simulink model "DataPath"  (R2025a)
settings: Solver=FixedStepAuto  StartTime=0  StopTime=0.02  FixedStep=1e-7  RelTol=1e-3
undefined symbols (not defined in the file): Bit_1, Bit_2, Bit_3, Bit_4, Bit_5, Bit_6, Bit_7, Bit_8
libraries: simulink_extras x126, fl_lib x34, nesl_utility x18, simulink x2
(part 4 of 7)

== system DataPath/Subsystem/ALU_REG/Subsystem1 ==
  Data : Inport
  Store : Inport  Port=2
  Clock : Inport  Port=3
  Clear : Inport  Port=4
  AND : Logic  IconShape=distinctive  AllPortsSameDT=off  OutDataTypeStr=boolean
  AND1 : Logic  IconShape=distinctive  AllPortsSameDT=off  OutDataTypeStr=boolean
  D Flip-Flop : simulink_extras/Flip Flops/D Flip-Flop
  NOT : Logic  Operator=NOT  IconShape=distinctive  AllPortsSameDT=off  OutDataTypeStr=boolean
  NOT1 : Logic  Operator=NOT  IconShape=distinctive  AllPortsSameDT=off  OutDataTypeStr=boolean
  OR : Logic  Operator=OR  IconShape=distinctive  AllPortsSameDT=off  OutDataTypeStr=boolean
  Q : Outport
  !Q : Outport  Port=2
  wires:
  AND1/1 -> OR/2
  AND/1 -> OR/1
  D Flip-Flop/1 -> Q/1, AND1/2
  NOT/1 -> AND1/1
  Store/1 -> AND/2, NOT/1
  Clock/1 -> D Flip-Flop/2
  Data/1 -> AND/1
  OR/1 -> D Flip-Flop/1
  D Flip-Flop/2 -> !Q/1
  Clear/1 -> NOT1/1
  NOT1/1 -> D Flip-Flop/3

== system DataPath/Subsystem/ALU_REG/Subsystem3 ==
  Data : Inport
  Store : Inport  Port=2
  Clock : Inport  Port=3
  Clear : Inport  Port=4
  AND : Logic  IconShape=distinctive  AllPortsSameDT=off  OutDataTypeStr=boolean
  AND1 : Logic  IconShape=distinctive  AllPortsSameDT=off  OutDataTypeStr=boolean
  D Flip-Flop : simulink_extras/Flip Flops/D Flip-Flop
  NOT : Logic  Operator=NOT  IconShape=distinctive  AllPortsSameDT=off  OutDataTypeStr=boolean
  NOT1 : Logic  Operator=NOT  IconShape=distinctive  AllPortsSameDT=off  OutDataTypeStr=boolean
  OR : Logic  Operator=OR  IconShape=distinctive  AllPortsSameDT=off  OutDataTypeStr=boolean
  Q : Outport
  !Q : Outport  Port=2
  wires:
  AND1/1 -> OR/2
  AND/1 -> OR/1
  D Flip-Flop/1 -> Q/1, AND1/2
  NOT/1 -> AND1/1
  Store/1 -> AND/2, NOT/1
  Clock/1 -> D Flip-Flop/2
  Data/1 -> AND/1
  OR/1 -> D Flip-Flop/1
  D Flip-Flop/2 -> !Q/1
  Clear/1 -> NOT1/1
  NOT1/1 -> D Flip-Flop/3

== system DataPath/Subsystem/Add Subtract Logic/Subsystem1 ==
  AND : Inport
  OR : Inport  Port=2
  XOR : Inport  Port=3
  !A : Inport  Port=4
  "!B " : Inport  Port=5
  SR : Inport  Port=6
  SL : Inport  Port=7
  OR1 : Logic  Operator=OR  Inputs=4  IconShape=distinctive  AllPortsSameDT=off  OutDataTypeStr=boolean
  OR2 : Logic  Operator=OR  Inputs=4  IconShape=distinctive  AllPortsSameDT=off  OutDataTypeStr=boolean
  OR3 : Logic  Operator=OR  Inputs=4  IconShape=distinctive  AllPortsSameDT=off  OutDataTypeStr=boolean
  C : Outport
  B : Outport  Port=2
  "A " : Outport  Port=3
  wires:
  OR2/1 -> C/1
  OR1/1 -> B/1
  OR3/1 -> "A "/1
  OR/1 -> OR3/1
  XOR/1 -> OR3/2, OR2/3
  !A/1 -> OR3/3, OR1/3
  "!B "/1 -> OR3/4, OR1/4, OR2/4
  SR/1 -> OR2/1
  SL/1 -> OR1/1
  AND/1 -> OR1/2, OR2/2

== system DataPath/Subsystem/Add Subtract Logic/Subsystem2 ==
  LO : Inport
  Enable : Inport  Port=2
  C : Inport  Port=3
  B : Inport  Port=4
  A : Inport  Port=5
  AND{6..17} (12 alike) : Logic  IconShape=distinctive  AllPortsSameDT=off  OutDataTypeStr=boolean
  NOT1 : Logic  Operator=NOT  IconShape=distinctive  AllPortsSameDT=off  OutDataTypeStr=boolean
  NOT2 : Logic  Operator=NOT  IconShape=distinctive  AllPortsSameDT=off  OutDataTypeStr=boolean
  NOT3 : Logic  Operator=NOT  IconShape=distinctive  AllPortsSameDT=off  OutDataTypeStr=boolean
  S-R Flip-Flop : simulink_extras/Flip Flops/S-R Flip-Flop  initial_condition=0
  S-R Flip-Flop1 : simulink_extras/Flip Flops/S-R Flip-Flop  initial_condition=0
  S-R Flip-Flop2 : simulink_extras/Flip Flops/S-R Flip-Flop  initial_condition=0
  A Stored : Outport
  B Stored : Outport  Port=2
  C Stored : Outport  Port=3
  wires:
  AND6/1 -> NOT3/1, AND14/2
  AND8/1 -> AND10/2, NOT1/1
  AND12/1 -> S-R Flip-Flop1/2
  NOT3/1 -> AND11/2
  Enable/1 -> AND8/1, AND7/1, AND6/1, AND13/1, AND12/1, AND11/1, AND10/1, AND9/1, AND14/1
  AND14/1 -> S-R Flip-Flop/1
  AND10/1 -> S-R Flip-Flop2/1
  S-R Flip-Flop1/1 -> AND16/1  "Data"
  AND7/1 -> AND9/2, NOT2/1
  AND11/1 -> S-R Flip-Flop/2
  B/1 -> AND7/2
  LO/1 -> AND17/2, AND16/2, AND15/2
  AND13/1 -> S-R Flip-Flop2/2
  AND17/1 -> C Stored/1
  A/1 -> AND6/2
  NOT2/1 -> AND12/2
  AND16/1 -> B Stored/1
  NOT1/1 -> AND13/2
  AND15/1 -> A Stored/1
  S-R Flip-Flop2/1 -> AND17/1  "Data"
  AND9/1 -> S-R Flip-Flop1/1
  S-R Flip-Flop/1 -> AND15/1  "Data"
  C/1 -> AND8/2

== system DataPath/Subsystem/Normalize Div/Subsystem1 ==
  Data : Inport
  CLK : Inport  Port=2
  NOT9 : Logic  Operator=NOT  IconShape=distinctive  AllPortsSameDT=off  OutDataTypeStr=boolean
  Subsystem6 : Subsystem
  Subsystem7 : Subsystem
  !Q : Outport
  Q : Outport  Port=2
  wires:
  Subsystem7/1(Q) -> Subsystem6/1(Data)
  Subsystem6/1(Q) -> Q/1
  CLK/1 -> Subsystem6/2(CLK), NOT9/1
  NOT9/1 -> Subsystem7/2(CLK)
  Data/1 -> Subsystem7/1(Data)
  Subsystem6/2(!Q) -> !Q/1

== system DataPath/Subsystem/Normalize Div/Subsystem8 ==
  Data : Inport
  CLK : Inport  Port=2
  NOT9 : Logic  Operator=NOT  IconShape=distinctive  AllPortsSameDT=off  OutDataTypeStr=boolean
  Subsystem6 : Subsystem
  Subsystem7 : Subsystem
  !Q : Outport
  Q : Outport  Port=2
  wires:
  Subsystem7/1(Q) -> Subsystem6/1(Data)
  Subsystem6/1(Q) -> Q/1
  NOT9/1 -> Subsystem7/2(CLK)
  Data/1 -> Subsystem7/1(Data)
  Subsystem6/2(!Q) -> !Q/1
  CLK/1 -> Subsystem6/2(CLK), NOT9/1

== system DataPath/Subsystem/Stepper/Subsystem1 ==
  "Step_{n-1}" : Inport
  CLK : Inport  Port=2
  "OR_{n+1}" : Inport  Port=3
  AND1 : Logic  IconShape=distinctive  AllPortsSameDT=off  OutDataTypeStr=boolean
  DFF : Subsystem
  Delay : Delay  DelayLength=1  InputProcessing=Columns as channels (frame based)  SampleTime=1e-6
  NOT1 : Logic  Operator=NOT  IconShape=distinctive  AllPortsSameDT=off  OutDataTypeStr=boolean
  OR1 : Logic  Operator=OR  IconShape=distinctive  AllPortsSameDT=off  OutDataTypeStr=boolean
  "Step_{n}" : Outport
  "!Step_{n}" : Outport  Port=2
  "OR_{n}" : Outport  Port=3
  wires:
  NOT1/1 -> "!Step_{n}"/1, AND1/2
  CLK/1 -> DFF/2(CLK)
  AND1/1 -> DFF/1(Data)
  "OR_{n+1}"/1 -> OR1/2
  "Step_{n-1}"/1 -> AND1/1
  DFF/1(Q) -> "Step_{n}"/1, OR1/1
  OR1/1 -> Delay/1
  Delay/1 -> "OR_{n}"/1, NOT1/1

== system DataPath/Subsystem/Stepper/Subsystem2 ==
  "Step_{n-1}" : Inport
  CLK : Inport  Port=2
  "OR_{n+1}" : Inport  Port=3
  AND1 : Logic  IconShape=distinctive  AllPortsSameDT=off  OutDataTypeStr=boolean
  DFF : Subsystem
  Delay : Delay  DelayLength=1  InputProcessing=Columns as channels (frame based)  SampleTime=1e-6
  Delay One Step : Delay  DelayLength=1
  Delay One Step1 : Delay  DelayLength=1
  NOT1 : Logic  Operator=NOT  IconShape=distinctive  AllPortsSameDT=off  OutDataTypeStr=boolean
  OR1 : Logic  Operator=OR  IconShape=distinctive  AllPortsSameDT=off  OutDataTypeStr=boolean
  "Step_{n}" : Outport
  "!Step_{n}" : Outport  Port=2
  "OR_{n}" : Outport  Port=3
  wires:
  Delay One Step1/1 -> "!Step_{n}"/1, AND1/2
  CLK/1 -> DFF/2(CLK)
  AND1/1 -> DFF/1(Data)
  "OR_{n+1}"/1 -> OR1/2
  "Step_{n-1}"/1 -> AND1/1
  DFF/1(Q) -> "Step_{n}"/1, OR1/1
  OR1/1 -> Delay/1
  Delay/1 -> Delay One Step/1, NOT1/1
  Delay One Step/1 -> "OR_{n}"/1
  NOT1/1 -> Delay One Step1/1

== system DataPath/Subsystem/Stepper/Subsystem3 ==
  "Step_{n-1}" : Inport
  CLK : Inport  Port=2
  "OR_{n+1}" : Inport  Port=3
  AND1 : Logic  IconShape=distinctive  AllPortsSameDT=off  OutDataTypeStr=boolean
  DFF : Subsystem
  Delay : Delay  DelayLength=1  InputProcessing=Columns as channels (frame based)  SampleTime=1e-6
  NOT1 : Logic  Operator=NOT  IconShape=distinctive  AllPortsSameDT=off  OutDataTypeStr=boolean
  OR1 : Logic  Operator=OR  IconShape=distinctive  AllPortsSameDT=off  OutDataTypeStr=boolean
  "Step_{n}" : Outport
  "!Step_{n}" : Outport  Port=2
  "OR_{n}" : Outport  Port=3
  wires:
  NOT1/1 -> "!Step_{n}"/1, AND1/2
  CLK/1 -> DFF/2(CLK)
  AND1/1 -> DFF/1(Data)
  "OR_{n+1}"/1 -> OR1/2
  "Step_{n-1}"/1 -> AND1/1
  DFF/1(Q) -> "Step_{n}"/1, OR1/1
  OR1/1 -> Delay/1
  Delay/1 -> "OR_{n}"/1, NOT1/1

== system DataPath/Subsystem/Stepper/Subsystem4 ==
  "Step_{n-1}" : Inport
  CLK : Inport  Port=2
  "OR_{n+1}" : Inport  Port=3
  AND1 : Logic  IconShape=distinctive  AllPortsSameDT=off  OutDataTypeStr=boolean
  DFF : Subsystem
  Delay : Delay  DelayLength=1  InputProcessing=Columns as channels (frame based)  SampleTime=1e-6
  NOT1 : Logic  Operator=NOT  IconShape=distinctive  AllPortsSameDT=off  OutDataTypeStr=boolean
  OR1 : Logic  Operator=OR  IconShape=distinctive  AllPortsSameDT=off  OutDataTypeStr=boolean
  "Step_{n}" : Outport
  "!Step_{n}" : Outport  Port=2
  "OR_{n}" : Outport  Port=3
  wires:
  NOT1/1 -> "!Step_{n}"/1, AND1/2
  CLK/1 -> DFF/2(CLK)
  AND1/1 -> DFF/1(Data)
  "OR_{n+1}"/1 -> OR1/2
  "Step_{n-1}"/1 -> AND1/1
  DFF/1(Q) -> "Step_{n}"/1, OR1/1
  OR1/1 -> Delay/1
  Delay/1 -> "OR_{n}"/1, NOT1/1

== system DataPath/Subsystem/Subsystem1/Subsystem ==
  Out A1-LO : Inport
  Out A1-Mult : Inport  Port=2
  Out A1-CD : Inport  Port=3
  Out A1-ND : Inport  Port=4
  Out A1-SDR : Inport  Port=5
  OR : Logic  Operator=OR  Inputs=5  IconShape=distinctive  AllPortsSameDT=off  OutDataTypeStr=boolean
  Out A1 : Outport
  wires:
  Out A1-LO/1 -> OR/5
  Out A1-Mult/1 -> OR/1
  OR/1 -> Out A1/1  "Out A1"
  Out A1-CD/1 -> OR/2
  Out A1-ND/1 -> OR/3
  Out A1-SDR/1 -> OR/4

== system DataPath/Subsystem/Subsystem1/Subsystem10 ==
  LSB-Mult : Inport
  LSB-CD : Inport  Port=2
  OR2 : Logic  Operator=OR  IconShape=distinctive  AllPortsSameDT=off  OutDataTypeStr=boolean
  LSB : Outport
  wires:
  LSB-CD/1 -> OR2/1
  LSB-Mult/1 -> OR2/2
  OR2/1 -> LSB/1  "LSB"

== system DataPath/Subsystem/Subsystem1/Subsystem11 ==
  NegA-ND : Inport
  NegA-SDR : Inport  Port=2
  OR1 : Logic  Operator=OR  IconShape=distinctive  AllPortsSameDT=off  OutDataTypeStr=boolean
  NegA : Outport
  wires:
  NegA-ND/1 -> OR1/1
  NegA-SDR/1 -> OR1/2
  OR1/1 -> NegA/1  "Bus Switch"

== system DataPath/Subsystem/Subsystem1/Subsystem13 ==
  Store B2-Mult : Inport
  Store B2-CD : Inport  Port=2
  Store B2-SDR : Inport  Port=3
  CLR : Inport  Port=4
  OR2 : Logic  Operator=OR  Inputs=4  IconShape=distinctive  AllPortsSameDT=off  OutDataTypeStr=boolean
  Store B2 : Outport
  wires:
  Store B2-CD/1 -> OR2/2
  OR2/1 -> Store B2/1  "Store B2"
  Store B2-SDR/1 -> OR2/3
  Store B2-Mult/1 -> OR2/1
  CLR/1 -> OR2/4

== system DataPath/Subsystem/Subsystem1/Subsystem14 ==
  Store B1-ICS : Inport
  Store B1-Mult : Inport  Port=2
  Store B1-ND : Inport  Port=3
  In4 : Inport  Port=4
  OR1 : Logic  Operator=OR  Inputs=4  IconShape=distinctive  AllPortsSameDT=off  OutDataTypeStr=boolean
  Store B1 : Outport
  wires:
  Store B1-ND/1 -> OR1/2
  Store B1-ICS/1 -> OR1/1
  OR1/1 -> Store B1/1  "Store B1"
  Store B1-Mult/1 -> OR1/3
  In4/1 -> OR1/4

== system DataPath/Subsystem/Subsystem1/Subsystem2 ==
  Out B2-Mult : Inport
  Out B2-CD : Inport  Port=2
  Out B2-SDR : Inport  Port=3
  OR2 : Logic  Operator=OR  Inputs=3  IconShape=distinctive  AllPortsSameDT=off  OutDataTypeStr=boolean
  Out B2 : Outport
  wires:
  Out B2-Mult/1 -> OR2/1
  Out B2-CD/1 -> OR2/2
  Out B2-SDR/1 -> OR2/3
  OR2/1 -> Out B2/1  "Out B2"

== system DataPath/Subsystem/Subsystem1/Subsystem3 ==
  Out ALU-LO : Inport
  Out ALU-Mult : Inport  Port=2
  Out ALU-ND : Inport  Port=3
  Out ALU-CD : Inport  Port=4
  Out ALU-SDR : Inport  Port=5
  OR3 : Logic  Operator=OR  Inputs=5  IconShape=distinctive  AllPortsSameDT=off  OutDataTypeStr=boolean
  Out ALU : Outport
  wires:
  Out ALU-SDR/1 -> OR3/4
  Out ALU-Mult/1 -> OR3/1
  OR3/1 -> Out ALU/1  "Out A1"
  Out ALU-LO/1 -> OR3/5
  Out ALU-ND/1 -> OR3/3
  Out ALU-CD/1 -> OR3/2

== system DataPath/Subsystem/Subsystem1/Subsystem5 ==
  Out B1-LO : Inport
  Out B1-mult : Inport  Port=2
  Out B1-CD : Inport  Port=3
  Out B1-ND : Inport  Port=4
  OR1 : Logic  Operator=OR  Inputs=4  IconShape=distinctive  AllPortsSameDT=off  OutDataTypeStr=boolean
  Out B1 : Outport
  wires:
  Out B1-CD/1 -> OR1/2
  Out B1-mult/1 -> OR1/1
  Out B1-LO/1 -> OR1/4
  OR1/1 -> Out B1/1  "Out B1"
  Out B1-ND/1 -> OR1/3

== system DataPath/Subsystem/Subsystem1/Subsystem6 ==
  Store A1-ICS : Inport
  Store A1-ND : Inport  Port=2
  Store A1-CD : Inport  Port=3
  Store A1-SDR : Inport  Port=4
  CLR : Inport  Port=5
  OR : Logic  Operator=OR  Inputs=5  IconShape=distinctive  AllPortsSameDT=off  OutDataTypeStr=boolean
  Store A1 : Outport
  wires:
  Store A1-CD/1 -> OR/2
  OR/1 -> Store A1/1  "Store A1"
  Store A1-ICS/1 -> OR/1
  Store A1-ND/1 -> OR/3
  Store A1-SDR/1 -> OR/4
  CLR/1 -> OR/5

== system DataPath/Subsystem/Subsystem1/Subsystem7 ==
  ADD ND : Inport
  ADD CD : Inport  Port=2
  ADD-SDR : Inport  Port=3
  OR1 : Logic  Operator=OR  Inputs=3  IconShape=distinctive  AllPortsSameDT=off  OutDataTypeStr=boolean
  "ADD " : Outport
  wires:
  ADD ND/1 -> OR1/2
  ADD CD/1 -> OR1/1
  OR1/1 -> "ADD "/1
  ADD-SDR/1 -> OR1/3

== system DataPath/Subsystem/Subsystem1/Subsystem9 ==
  Out DP-LO : Inport
  Out DP-Mult : Inport  Port=2
  Out DP-Div : Inport  Port=3
  OR3 : Logic  Operator=OR  Inputs=3  IconShape=distinctive  AllPortsSameDT=off  OutDataTypeStr=boolean
  Out DP : Outport
  wires:
  OR3/1 -> Out DP/1
  Out DP-Mult/1 -> OR3/2
  Out DP-Div/1 -> OR3/3
  Out DP-LO/1 -> OR3/1

== system DataPath/Subsystem1/ALU/ALU MUX ==
  note: Each Enabler is a set of 8 tri-state buffers
  0/0/0 : Inport
  0/0/1 : Inport  Port=2
  0/1/0 : Inport  Port=3
  0/1/1 : Inport  Port=4
  1/0/0 : Inport  Port=5
  1/0/1 : Inport  Port=6
  1/1/0 : Inport  Port=7
  1/1/1 : Inport  Port=8
  Bus1 : Inport  Port=9
  Bus2 : Inport  Port=10
  Bus3 : Inport  Port=11
  Bus4 : Inport  Port=12
  Bus5 : Inport  Port=13
  Bus6 : Inport  Port=14
  Bus7 : Inport  Port=15
  Bus8 : Inport  Port=16
  Delay One Step1 : Delay  DelayLength=1
  Delay One Step3 : Delay  DelayLength=1
  MATLAB Function1 : MATLAB Function  TreatAsAtomicUnit=on
  MATLAB Function2 : MATLAB Function  TreatAsAtomicUnit=on
  MATLAB Function3 : MATLAB Function  TreatAsAtomicUnit=on
  MATLAB Function4 : MATLAB Function  TreatAsAtomicUnit=on
  MATLAB Function5 : MATLAB Function  TreatAsAtomicUnit=on
  MATLAB Function6 : MATLAB Function  TreatAsAtomicUnit=on
  MATLAB Function7 : MATLAB Function  TreatAsAtomicUnit=on
  MATLAB Function8 : MATLAB Function  TreatAsAtomicUnit=on
  Mux : Mux  Inputs=8
  Mux1 : Mux  Inputs=8
  ALU Output : Outport
  wires:
  1/1/1/1 -> Mux/8
  1/1/0/1 -> Mux/7
  1/0/1/1 -> Mux/6
  1/0/0/1 -> Mux/5
  0/1/1/1 -> Mux/4
  0/1/0/1 -> Mux/3
  0/0/1/1 -> Mux/2
  0/0/0/1 -> Mux/1
  Bus3/1 -> MATLAB Function2/1(InputBus)
  Bus5/1 -> MATLAB Function4/1(InputBus)
  Bus8/1 -> MATLAB Function8/1(InputBus)
  Bus2/1 -> MATLAB Function6/1(InputBus)
  Bus4/1 -> MATLAB Function3/1(InputBus)
  Bus1/1 -> MATLAB Function1/1(InputBus)
  Bus6/1 -> MATLAB Function5/1(InputBus)
  Bus7/1 -> MATLAB Function7/1(InputBus)
  Mux/1 -> MATLAB Function8/2(Selection), MATLAB Function7/2(Selection), MATLAB Function5/2(Selection), MATLAB Function4/2(Selection), MATLAB Function3/2(Selection), MATLAB Function2/2(Selection), MATLAB Function1/2(Selection), MATLAB Function6/2(Selection)
  MATLAB Function6/1(output) -> Mux1/2
  MATLAB Function2/1(output) -> Mux1/3
  MATLAB Function3/1(output) -> Mux1/4
  MATLAB Function4/1(output) -> Mux1/5
  MATLAB Function5/1(output) -> Mux1/6
  MATLAB Function7/1(output) -> Mux1/7
  MATLAB Function8/1(output) -> Mux1/8
  MATLAB Function1/1(output) -> Mux1/1
  Mux1/1 -> Delay One Step1/1
  Delay One Step1/1 -> ALU Output/1

== system DataPath/Subsystem1/ALU/Adder & Logic Module ==
  Subtract mode : Inport
  Neg_A : Inport  Port=2
  Bus_A : Inport  Port=3
  Bus_B : Inport  Port=4
  Constant : Constant
  Constant1 : Constant  Value=0
  Delay One Step1 : Delay  DelayLength=1
  Delay One Step3 : Delay  DelayLength=1
  Demux1 : Demux  Outputs=8
  Demux2 : Demux  Outputs=8
  Display1 : Display
  Display3 : Display
  MATLAB Function1 : MATLAB Function  TreatAsAtomicUnit=on
  MATLAB Function3 : MATLAB Function  TreatAsAtomicUnit=on
  Subsystem1 : Subsystem
      settings: PortSchema="{\"entries\":[{\"content\":{\"sides\":[{\"content\":{\"connectorIds\":[\"In1\",\"In2\",\"Out3\",\"Out4\"]},\"type\":\"ConnectorPlacement.EquallySpacedRectSide\",\"uuid\":\"d566efe6-1fc5-4e96-a6c3-64a47f89d9c9\"},{\"content\":{\"connectorIds\":[\"Out1\",\"In6\",\"In7\"],\"side\":\"RIGHT\"},\"type\":\"ConnectorPlacement.EquallySpacedRectSide\",\"uuid\":\"006cd780-973d-4bae-abc8-89f745b28566\"},{\"content\":{\"connectorIds\":[\"In3\",\"In4\"],\"side\":\"TOP\"},\"type\":\"ConnectorPlacement.EquallySpacedRectSide\",\"uuid\":\"c760ecb1-3a5c-4ba0-9224-1c9b5ce710fd\"},{\"content\":{\"connectorIds\":[\"In5\",\"Out2\"],\"side\":\"BOTTOM\"},\"type\":\"ConnectorPlacement.EquallySpacedRectSide\",\"uuid\":\"178f6c5d-529f-4f0d-80ca-fb6729cf398e\"}]},\"type\":\"ConnectorPlacement.EquallySpacedConnector\",\"uuid\":\"d5293939-72db-46a2-88f3-163e4f70d202\"}],\"packageUris\":[\"http://schema.mathworks.com/mf0/Connector/R2020b\"],\"version\":\"1.0\"}"
  Subsystem2 : Subsystem
      settings: PortSchema="{\"entries\":[{\"content\":{\"sides\":[{\"content\":{\"connectorIds\":[\"In1\",\"In2\",\"Out3\",\"Out4\"]},\"type\":\"ConnectorPlacement.EquallySpacedRectSide\",\"uuid\":\"d566efe6-1fc5-4e96-a6c3-64a47f89d9c9\"},{\"content\":{\"connectorIds\":[\"Out1\",\"In6\",\"In7\"],\"side\":\"RIGHT\"},\"type\":\"ConnectorPlacement.EquallySpacedRectSide\",\"uuid\":\"006cd780-973d-4bae-abc8-89f745b28566\"},{\"content\":{\"connectorIds\":[\"In3\",\"In4\"],\"side\":\"TOP\"},\"type\":\"ConnectorPlacement.EquallySpacedRectSide\",\"uuid\":\"c760ecb1-3a5c-4ba0-9224-1c9b5ce710fd\"},{\"content\":{\"connectorIds\":[\"In5\",\"Out2\"],\"side\":\"BOTTOM\"},\"type\":\"ConnectorPlacement.EquallySpacedRectSide\",\"uuid\":\"178f6c5d-529f-4f0d-80ca-fb6729cf398e\"}]},\"type\":\"ConnectorPlacement.EquallySpacedConnector\",\"uuid\":\"d5293939-72db-46a2-88f3-163e4f70d202\"}],\"packageUris\":[\"http://schema.mathworks.com/mf0/Connector/R2020b\"],\"version\":\"1.0\"}"
  Subsystem3 : Subsystem
      settings: PortSchema="{\"entries\":[{\"content\":{\"sides\":[{\"content\":{\"connectorIds\":[\"In1\",\"In2\",\"Out3\",\"Out4\"]},\"type\":\"ConnectorPlacement.EquallySpacedRectSide\",\"uuid\":\"d566efe6-1fc5-4e96-a6c3-64a47f89d9c9\"},{\"content\":{\"connectorIds\":[\"Out1\",\"In6\",\"In7\"],\"side\":\"RIGHT\"},\"type\":\"ConnectorPlacement.EquallySpacedRectSide\",\"uuid\":\"006cd780-973d-4bae-abc8-89f745b28566\"},{\"content\":{\"connectorIds\":[\"In3\",\"In4\"],\"side\":\"TOP\"},\"type\":\"ConnectorPlacement.EquallySpacedRectSide\",\"uuid\":\"c760ecb1-3a5c-4ba0-9224-1c9b5ce710fd\"},{\"content\":{\"connectorIds\":[\"In5\",\"Out2\"],\"side\":\"BOTTOM\"},\"type\":\"ConnectorPlacement.EquallySpacedRectSide\",\"uuid\":\"178f6c5d-529f-4f0d-80ca-fb6729cf398e\"}]},\"type\":\"ConnectorPlacement.EquallySpacedConnector\",\"uuid\":\"d5293939-72db-46a2-88f3-163e4f70d202\"}],\"packageUris\":[\"http://schema.mathworks.com/mf0/Connector/R2020b\"],\"version\":\"1.0\"}"
  Subsystem4 : Subsystem
      settings: PortSchema="{\"entries\":[{\"content\":{\"sides\":[{\"content\":{\"connectorIds\":[\"In1\",\"In2\",\"Out3\",\"Out4\"]},\"type\":\"ConnectorPlacement.EquallySpacedRectSide\",\"uuid\":\"d566efe6-1fc5-4e96-a6c3-64a47f89d9c9\"},{\"content\":{\"connectorIds\":[\"Out1\",\"In6\",\"In7\"],\"side\":\"RIGHT\"},\"type\":\"ConnectorPlacement.EquallySpacedRectSide\",\"uuid\":\"006cd780-973d-4bae-abc8-89f745b28566\"},{\"content\":{\"connectorIds\":[\"In3\",\"In4\"],\"side\":\"TOP\"},\"type\":\"ConnectorPlacement.EquallySpacedRectSide\",\"uuid\":\"c760ecb1-3a5c-4ba0-9224-1c9b5ce710fd\"},{\"content\":{\"connectorIds\":[\"In5\",\"Out2\"],\"side\":\"BOTTOM\"},\"type\":\"ConnectorPlacement.EquallySpacedRectSide\",\"uuid\":\"178f6c5d-529f-4f0d-80ca-fb6729cf398e\"}]},\"type\":\"ConnectorPlacement.EquallySpacedConnector\",\"uuid\":\"d5293939-72db-46a2-88f3-163e4f70d202\"}],\"packageUris\":[\"http://schema.mathworks.com/mf0/Connector/R2020b\"],\"version\":\"1.0\"}"
  Subsystem5 : Subsystem
      settings: PortSchema="{\"entries\":[{\"content\":{\"sides\":[{\"content\":{\"connectorIds\":[\"In1\",\"In2\",\"Out3\",\"Out4\"]},\"type\":\"ConnectorPlacement.EquallySpacedRectSide\",\"uuid\":\"d566efe6-1fc5-4e96-a6c3-64a47f89d9c9\"},{\"content\":{\"connectorIds\":[\"Out1\",\"In6\",\"In7\"],\"side\":\"RIGHT\"},\"type\":\"ConnectorPlacement.EquallySpacedRectSide\",\"uuid\":\"006cd780-973d-4bae-abc8-89f745b28566\"},{\"content\":{\"connectorIds\":[\"In3\",\"In4\"],\"side\":\"TOP\"},\"type\":\"ConnectorPlacement.EquallySpacedRectSide\",\"uuid\":\"c760ecb1-3a5c-4ba0-9224-1c9b5ce710fd\"},{\"content\":{\"connectorIds\":[\"In5\",\"Out2\"],\"side\":\"BOTTOM\"},\"type\":\"ConnectorPlacement.EquallySpacedRectSide\",\"uuid\":\"178f6c5d-529f-4f0d-80ca-fb6729cf398e\"}]},\"type\":\"ConnectorPlacement.EquallySpacedConnector\",\"uuid\":\"d5293939-72db-46a2-88f3-163e4f70d202\"}],\"packageUris\":[\"http://schema.mathworks.com/mf0/Connector/R2020b\"],\"version\":\"1.0\"}"
  Subsystem6 : Subsystem
      settings: PortSchema="{\"entries\":[{\"content\":{\"sides\":[{\"content\":{\"connectorIds\":[\"In1\",\"In2\",\"Out3\",\"Out4\"]},\"type\":\"ConnectorPlacement.EquallySpacedRectSide\",\"uuid\":\"d566efe6-1fc5-4e96-a6c3-64a47f89d9c9\"},{\"content\":{\"connectorIds\":[\"Out1\",\"In6\",\"In7\"],\"side\":\"RIGHT\"},\"type\":\"ConnectorPlacement.EquallySpacedRectSide\",\"uuid\":\"006cd780-973d-4bae-abc8-89f745b28566\"},{\"content\":{\"connectorIds\":[\"In3\",\"In4\"],\"side\":\"TOP\"},\"type\":\"ConnectorPlacement.EquallySpacedRectSide\",\"uuid\":\"c760ecb1-3a5c-4ba0-9224-1c9b5ce710fd\"},{\"content\":{\"connectorIds\":[\"In5\",\"Out2\"],\"side\":\"BOTTOM\"},\"type\":\"ConnectorPlacement.EquallySpacedRectSide\",\"uuid\":\"178f6c5d-529f-4f0d-80ca-fb6729cf398e\"}]},\"type\":\"ConnectorPlacement.EquallySpacedConnector\",\"uuid\":\"d5293939-72db-46a2-88f3-163e4f70d202\"}],\"packageUris\":[\"http://schema.mathworks.com/mf0/Connector/R2020b\"],\"version\":\"1.0\"}"
  Subsystem7 : Subsystem
      settings: PortSchema="{\"entries\":[{\"content\":{\"sides\":[{\"content\":{\"connectorIds\":[\"In1\",\"In2\",\"Out3\",\"Out4\"]},\"type\":\"ConnectorPlacement.EquallySpacedRectSide\",\"uuid\":\"d566efe6-1fc5-4e96-a6c3-64a47f89d9c9\"},{\"content\":{\"connectorIds\":[\"Out1\",\"In6\",\"In7\"],\"side\":\"RIGHT\"},\"type\":\"ConnectorPlacement.EquallySpacedRectSide\",\"uuid\":\"006cd780-973d-4bae-abc8-89f745b28566\"},{\"content\":{\"connectorIds\":[\"In3\",\"In4\"],\"side\":\"TOP\"},\"type\":\"ConnectorPlacement.EquallySpacedRectSide\",\"uuid\":\"c760ecb1-3a5c-4ba0-9224-1c9b5ce710fd\"},{\"content\":{\"connectorIds\":[\"In5\",\"Out2\"],\"side\":\"BOTTOM\"},\"type\":\"ConnectorPlacement.EquallySpacedRectSide\",\"uuid\":\"178f6c5d-529f-4f0d-80ca-fb6729cf398e\"}]},\"type\":\"ConnectorPlacement.EquallySpacedConnector\",\"uuid\":\"d5293939-72db-46a2-88f3-163e4f70d202\"}],\"packageUris\":[\"http://schema.mathworks.com/mf0/Connector/R2020b\"],\"version\":\"1.0\"}"
  Subsystem8 : Subsystem
      settings: PortSchema="{\"entries\":[{\"content\":{\"sides\":[{\"content\":{\"connectorIds\":[\"In1\",\"In2\",\"Out3\",\"Out4\"]},\"type\":\"ConnectorPlacement.EquallySpacedRectSide\",\"uuid\":\"d566efe6-1fc5-4e96-a6c3-64a47f89d9c9\"},{\"content\":{\"connectorIds\":[\"Out1\",\"In6\",\"In7\"],\"side\":\"RIGHT\"},\"type\":\"ConnectorPlacement.EquallySpacedRectSide\",\"uuid\":\"006cd780-973d-4bae-abc8-89f745b28566\"},{\"content\":{\"connectorIds\":[\"In3\",\"In4\"],\"side\":\"TOP\"},\"type\":\"ConnectorPlacement.EquallySpacedRectSide\",\"uuid\":\"c760ecb1-3a5c-4ba0-9224-1c9b5ce710fd\"},{\"content\":{\"connectorIds\":[\"In5\",\"Out2\"],\"side\":\"BOTTOM\"},\"type\":\"ConnectorPlacement.EquallySpacedRectSide\",\"uuid\":\"178f6c5d-529f-4f0d-80ca-fb6729cf398e\"}]},\"type\":\"ConnectorPlacement.EquallySpacedConnector\",\"uuid\":\"d5293939-72db-46a2-88f3-163e4f70d202\"}],\"packageUris\":[\"http://schema.mathworks.com/mf0/Connector/R2020b\"],\"version\":\"1.0\"}"
  Bus1 : Outport
  Bus2 : Outport  Port=2
  Bus3 : Outport  Port=3
  Bus4 : Outport  Port=4
  Bus5 : Outport  Port=5
  Bus6 : Outport  Port=6
  Bus7 : Outport  Port=7
  Bus8 : Outport  Port=8
  A=B : Outport  Port=9
  A>B : Outport  Port=10
  Overflow : Outport  Port=11
  wires:
  Subsystem8/1(Carry Out) -> Subsystem2/2(Carry In)
  Subsystem6/1(Carry Out) -> Subsystem5/2(Carry In)
  Subsystem3/1(Carry Out) -> Subsystem6/2(Carry In)
  Subsystem8/2(Bus) -> Bus8/1
  Subsystem7/2(Bus) -> Bus1/1
  Subsystem4/2(Bus) -> Bus2/1
  Subsystem5/2(Bus) -> Bus3/1
  Subsystem6/2(Bus) -> Bus4/1
  Subsystem3/2(Bus) -> Bus5/1
  Subsystem1/2(Bus) -> Bus6/1
  Subsystem2/2(Bus) -> Bus7/1
  Subtract mode/1 -> Subsystem8/2(Carry In), Subsystem8/5(Subtract), Subsystem7/5(Subtract), Subsystem2/5(Subtract), Subsystem4/5(Subtract), Subsystem1/5(Subtract), Subsystem5/5(Subtract), Subsystem6/5(Subtract), Subsystem3/5(Subtract)
  Subsystem7/1(Carry Out) -> Overflow/1
  Bus_A/1 -> Delay One Step3/1  "Bus A"
  MATLAB Function1/1(Decimal) -> Display1/1
  Bus_B/1 -> Delay One Step1/1  "Bus B"
  MATLAB Function3/1(Decimal) -> Display3/1
  Subsystem2/1(Carry Out) -> Subsystem1/2(Carry In)
  Subsystem1/1(Carry Out) -> Subsystem3/2(Carry In)
  Subsystem5/1(Carry Out) -> Subsystem4/2(Carry In)
  Subsystem4/1(Carry Out) -> Subsystem7/2(Carry In)
  Neg_A/1 -> Subsystem8/1(Neg_A), Subsystem2/1(Neg_A), Subsystem1/1(Neg_A), Subsystem6/1(Neg_A), Subsystem5/1(Neg_A), Subsystem4/1(Neg_A), Subsystem7/1(Neg_A), Subsystem3/1(Neg_A)
  Delay One Step3/1 -> MATLAB Function1/1(Binary), Demux2/1
  Delay One Step1/1 -> MATLAB Function3/1(Binary), Demux1/1
  Demux1/1 -> Subsystem7/3(B)
  Demux1/2 -> Subsystem4/3(B)
  Demux1/3 -> Subsystem5/3(B)
  Demux1/4 -> Subsystem6/3(B)
  Demux1/5 -> Subsystem3/3(B)
  Demux1/6 -> Subsystem1/3(B)
  Demux1/7 -> Subsystem2/3(B)
  Demux1/8 -> Subsystem8/3(B)
  Demux2/8 -> Subsystem8/4(A)
  Demux2/7 -> Subsystem2/4(A)
  Demux2/6 -> Subsystem1/4(A)
  Demux2/5 -> Subsystem3/4(A)
  Demux2/4 -> Subsystem6/4(A)
  Demux2/3 -> Subsystem5/4(A)
  Demux2/2 -> Subsystem4/4(A)
  Demux2/1 -> Subsystem7/4(A)
  Subsystem7/3(A >B Next) -> Subsystem4/6(A>B Prev)
  Subsystem7/4(= Currently) -> Subsystem4/7(= So far)
  Subsystem4/4(= Currently) -> Subsystem5/7(= So far)
  Subsystem4/3(A >B Next) -> Subsystem5/6(A>B Prev)
  Subsystem5/4(= Currently) -> Subsystem6/7(= So far)
  Subsystem5/3(A >B Next) -> Subsystem6/6(A>B Prev)
  Constant/1 -> Subsystem7/7(= So far)
  Subsystem1/3(= Currently) -> Subsystem2/6(= So far)
  Subsystem1/4(A >B Next) -> Subsystem2/7(A>B Prev)
  Subsystem3/4(A >B Next) -> Subsystem1/7(A>B Prev)
  Subsystem3/3(= Currently) -> Subsystem1/6(= So far)
  Subsystem2/4(A >B Next) -> Subsystem8/7(A>B Prev)
  Subsystem2/3(= Currently) -> Subsystem8/6(= So far)
  Subsystem8/4(A >B Next) -> A>B/1
  Subsystem8/3(= Currently) -> A=B/1
  Subsystem6/4(= Currently) -> Subsystem3/6(= So far)
  Subsystem6/3(A >B Next) -> Subsystem3/7(A>B Prev)
  Constant1/1 -> Subsystem7/6(A>B Prev)

== system DataPath/Subsystem1/ALU/FlagAndDecode ==
  note: A/B/C
  SM : Inport
  Sel_A : Inport  Port=2
  Sel_B : Inport  Port=3
  Sel_C : Inport  Port=4
  ALU Bus : Inport  Port=5
  Overflow : Inport  Port=6
  AND1 : Logic  IconShape=distinctive  AllPortsSameDT=off  OutDataTypeStr=boolean
  AND{3..10} (8 alike) : Logic  Inputs=3  IconShape=distinctive  AllPortsSameDT=off  OutDataTypeStr=boolean
  AND2 : Logic  IconShape=distinctive  AllPortsSameDT=off  OutDataTypeStr=boolean
  Demux1 : Demux  Outputs=8
  NAND : Logic  Operator=NAND  IconShape=distinctive  AllPortsSameDT=off  OutDataTypeStr=boolean
  NOR1 : Logic  Operator=NOR  Inputs=8  IconShape=distinctive  AllPortsSameDT=off  OutDataTypeStr=boolean
  NOT{,1..3} (4 alike) : Logic  Operator=NOT  IconShape=distinctive  AllPortsSameDT=off  OutDataTypeStr=boolean
  0/0/0 : Outport
  0/0/1 : Outport  Port=2
  0/1/0 : Outport  Port=3
  0/1/1 : Outport  Port=4
  1/0/0 : Outport  Port=5
  1/0/1 : Outport  Port=6
  1/1/0 : Outport  Port=7
  1/1/1 : Outport  Port=8
  Zero : Outport  Port=9
  Negative : Outport  Port=10
  wires:
  SM/1 -> AND2/1, NOT/1
  Demux1/1 -> NOR1/1, AND2/2
  NOT/1 -> NAND/2
  Demux1/4 -> NOR1/4
  NOR1/1 -> AND1/2  "Byte_zero"
  Overflow/1 -> NAND/1
  Demux1/5 -> NOR1/5
  NAND/1 -> AND1/1  "No_Overflow"
  Demux1/8 -> NOR1/8
  Demux1/6 -> NOR1/6
  ALU Bus/1 -> Demux1/1
  Demux1/7 -> NOR1/7
  Demux1/3 -> NOR1/3
  AND1/1 -> Zero/1  "Zero"
  AND2/1 -> Negative/1
  Demux1/2 -> NOR1/2
  AND3/1 -> 0/0/0/1
  NOT1/1 -> AND6/1, AND5/1, AND4/1, AND3/1
  AND9/1 -> 1/1/0/1
  Sel_C/1 -> AND10/3, AND8/3, AND6/3, AND4/3, NOT3/1
  AND7/1 -> 1/0/0/1
  AND6/1 -> 0/1/1/1
  NOT2/1 -> AND4/2, AND7/2, AND8/2, AND3/2
  Sel_B/1 -> AND10/2, AND9/2, AND6/2, AND5/2, NOT2/1
  AND4/1 -> 0/0/1/1
  NOT3/1 -> AND9/3, AND7/3, AND5/3, AND3/3
  Sel_A/1 -> AND10/1, AND9/1, AND8/1, AND7/1, NOT1/1
  AND5/1 -> 0/1/0/1
  AND8/1 -> 1/0/1/1
  AND10/1 -> 1/1/1/1

== system DataPath/Subsystem1/ALU Regs/A1 ==
  Data bus : Inport
  Store : Inport  Port=2
  CLK : Inport  Port=3
  Demux : Demux  Outputs=8
  Mux : Mux  Inputs=8
  Subsystem1 : Subsystem
  Subsystem2 : Subsystem
  Subsystem3 : Subsystem
  Subsystem4 : Subsystem
  Subsystem5 : Subsystem
  Subsystem6 : Subsystem
  Subsystem7 : Subsystem
  Subsystem8 : Subsystem
  "Q Bus " : Outport
  wires:
  Demux/4 -> Subsystem2/1(Data)
  Mux/1 -> "Q Bus "/1
  Demux/2 -> Subsystem1/1(Data)
  Data bus/1 -> Demux/1
  Subsystem6/1(Q) -> Mux/8
  Store/1 -> Subsystem1/2(Store), Subsystem4/2(Store), Subsystem2/2(Store), Subsystem7/2(Store), Subsystem5/2(Store), Subsystem6/2(Store), Subsystem8/2(Store), Subsystem3/2(Store)
  Demux/5 -> Subsystem7/1(Data)
  Demux/7 -> Subsystem8/1(Data)
  Demux/3 -> Subsystem4/1(Data)
  Subsystem7/1(Q) -> Mux/5
  Demux/6 -> Subsystem5/1(Data)
  Subsystem1/1(Q) -> Mux/2
  Demux/1 -> Subsystem3/1(Data)
  Subsystem3/1(Q) -> Mux/1
  Demux/8 -> Subsystem6/1(Data)
  Subsystem8/1(Q) -> Mux/7
  Subsystem2/1(Q) -> Mux/4
  Subsystem4/1(Q) -> Mux/3
  Subsystem5/1(Q) -> Mux/6
  CLK/1 -> Subsystem1/3(Clock), Subsystem4/3(Clock), Subsystem2/3(Clock), Subsystem7/3(Clock), Subsystem5/3(Clock), Subsystem6/3(Clock), Subsystem8/3(Clock), Subsystem3/3(Clock)

== system DataPath/Subsystem1/ALU Regs/A2 ==
  Data bus : Inport
  Store : Inport  Port=2
  CLK : Inport  Port=3
  Demux : Demux  Outputs=8
  Mux : Mux  Inputs=8
  Subsystem1 : Subsystem
  Subsystem2 : Subsystem
  Subsystem3 : Subsystem
  Subsystem4 : Subsystem
  Subsystem5 : Subsystem
  Subsystem6 : Subsystem
  Subsystem7 : Subsystem
  Subsystem8 : Subsystem
  "Q Bus " : Outport
  wires:
  Demux/4 -> Subsystem2/1(Data)
  Mux/1 -> "Q Bus "/1
  Demux/2 -> Subsystem1/1(Data)
  Data bus/1 -> Demux/1
  Subsystem6/1(Q) -> Mux/8
  Store/1 -> Subsystem1/2(Store), Subsystem4/2(Store), Subsystem2/2(Store), Subsystem7/2(Store), Subsystem5/2(Store), Subsystem6/2(Store), Subsystem8/2(Store), Subsystem3/2(Store)
  Demux/5 -> Subsystem7/1(Data)
  Demux/7 -> Subsystem8/1(Data)
  Demux/3 -> Subsystem4/1(Data)
  Subsystem7/1(Q) -> Mux/5
  Demux/6 -> Subsystem5/1(Data)
  Subsystem1/1(Q) -> Mux/2
  Demux/1 -> Subsystem3/1(Data)
  Subsystem3/1(Q) -> Mux/1
  Demux/8 -> Subsystem6/1(Data)
  Subsystem8/1(Q) -> Mux/7
  Subsystem2/1(Q) -> Mux/4
  Subsystem4/1(Q) -> Mux/3
  Subsystem5/1(Q) -> Mux/6
  CLK/1 -> Subsystem1/3(Clock), Subsystem4/3(Clock), Subsystem2/3(Clock), Subsystem7/3(Clock), Subsystem5/3(Clock), Subsystem6/3(Clock), Subsystem8/3(Clock), Subsystem3/3(Clock)

== system DataPath/Subsystem1/ALU Regs/B1 ==
  Data bus : Inport
  Store : Inport  Port=2
  CLK : Inport  Port=3
  Demux : Demux  Outputs=8
  Mux : Mux  Inputs=8
  Subsystem1 : Subsystem
  Subsystem2 : Subsystem
  Subsystem3 : Subsystem
  Subsystem4 : Subsystem
  Subsystem5 : Subsystem
  Subsystem6 : Subsystem
  Subsystem7 : Subsystem
  Subsystem8 : Subsystem
  "Q Bus " : Outport
  wires:
  Demux/4 -> Subsystem2/1(Data)
  Mux/1 -> "Q Bus "/1
  Demux/2 -> Subsystem1/1(Data)
  Data bus/1 -> Demux/1
  Subsystem6/1(Q) -> Mux/8
  Store/1 -> Subsystem1/2(Store), Subsystem4/2(Store), Subsystem2/2(Store), Subsystem7/2(Store), Subsystem5/2(Store), Subsystem6/2(Store), Subsystem8/2(Store), Subsystem3/2(Store)
  Demux/5 -> Subsystem7/1(Data)
  Demux/7 -> Subsystem8/1(Data)
  Demux/3 -> Subsystem4/1(Data)
  Subsystem7/1(Q) -> Mux/5
  Demux/6 -> Subsystem5/1(Data)
  Subsystem1/1(Q) -> Mux/2
  Demux/1 -> Subsystem3/1(Data)
  Subsystem3/1(Q) -> Mux/1
  Demux/8 -> Subsystem6/1(Data)
  Subsystem8/1(Q) -> Mux/7
  Subsystem2/1(Q) -> Mux/4
  Subsystem4/1(Q) -> Mux/3
  Subsystem5/1(Q) -> Mux/6
  CLK/1 -> Subsystem1/3(Clock), Subsystem4/3(Clock), Subsystem2/3(Clock), Subsystem7/3(Clock), Subsystem5/3(Clock), Subsystem6/3(Clock), Subsystem8/3(Clock), Subsystem3/3(Clock)

== system DataPath/Subsystem1/ALU Regs/B2 ==
  Data bus : Inport
  Store : Inport  Port=2
  CLK : Inport  Port=3
  Demux : Demux  Outputs=8
  Mux : Mux  Inputs=8
  Subsystem1 : Subsystem
  Subsystem2 : Subsystem
  Subsystem3 : Subsystem
  Subsystem4 : Subsystem
  Subsystem5 : Subsystem
  Subsystem6 : Subsystem
  Subsystem7 : Subsystem
  Subsystem8 : Subsystem
  "Q Bus " : Outport
  wires:
  Demux/4 -> Subsystem2/1(Data)
  Mux/1 -> "Q Bus "/1
  Demux/2 -> Subsystem1/1(Data)
  Data bus/1 -> Demux/1
  Subsystem6/1(Q) -> Mux/8
  Store/1 -> Subsystem1/2(Store), Subsystem4/2(Store), Subsystem2/2(Store), Subsystem7/2(Store), Subsystem5/2(Store), Subsystem6/2(Store), Subsystem8/2(Store), Subsystem3/2(Store)
  Demux/5 -> Subsystem7/1(Data)
  Demux/7 -> Subsystem8/1(Data)
  Demux/3 -> Subsystem4/1(Data)
  Subsystem7/1(Q) -> Mux/5
  Demux/6 -> Subsystem5/1(Data)
  Subsystem1/1(Q) -> Mux/2
  Demux/1 -> Subsystem3/1(Data)
  Subsystem3/1(Q) -> Mux/1
  Demux/8 -> Subsystem6/1(Data)
  Subsystem8/1(Q) -> Mux/7
  Subsystem2/1(Q) -> Mux/4
  Subsystem4/1(Q) -> Mux/3
  Subsystem5/1(Q) -> Mux/6
  CLK/1 -> Subsystem1/3(Clock), Subsystem4/3(Clock), Subsystem2/3(Clock), Subsystem7/3(Clock), Subsystem5/3(Clock), Subsystem6/3(Clock), Subsystem8/3(Clock), Subsystem3/3(Clock)

== system DataPath/Subsystem1/ALU Regs/Subsystem2 ==
  Bus B1 : Inport
  B1 : Inport  Port=2
  B2 : Inport  Port=3
  Bus B 2 : Inport  Port=4
  Demux : Demux  Outputs=8
  Demux1 : Demux  Outputs=8
  MATLAB Function : MATLAB Function  TreatAsAtomicUnit=on
  Multiport Switch{,1..7} (8 alike) : MultiPortSwitch  DataPortOrder=Specify indices  Inputs=2  DataPortIndices={0,1,-1}  SaturateOnIntegerOverflow=off  InputSameDT=off
  Mux : Mux  Inputs=8
  Zero{,1..7} (8 alike) : Constant  Value=0  OutDataTypeStr=Inherit: Inherit via back propagation
  But Out : Outport
  wires:
  Demux1/7 -> Multiport Switch6/3
  Multiport Switch2/1 -> Mux/3
  Demux/4 -> Multiport Switch3/2
  Bus B 2/1 -> Demux1/1
  Multiport Switch6/1 -> Mux/7
  Demux1/1 -> Multiport Switch/3
  Multiport Switch3/1 -> Mux/4
  Zero/1 -> Multiport Switch/4
  MATLAB Function/1(Select) -> Multiport Switch7/1, Multiport Switch6/1, Multiport Switch5/1, Multiport Switch4/1, Multiport Switch3/1, Multiport Switch2/1, Multiport Switch1/1, Multiport Switch/1
  Demux/2 -> Multiport Switch1/2
  Demux/6 -> Multiport Switch5/2
  Demux/8 -> Multiport Switch7/2
  Multiport Switch/1 -> Mux/1
  Demux1/3 -> Multiport Switch2/3
  Zero6/1 -> Multiport Switch6/4
  Bus B1/1 -> Demux/1
  B2/1 -> MATLAB Function/2(A2)
  Zero5/1 -> Multiport Switch5/4
  Zero4/1 -> Multiport Switch4/4
  Demux/5 -> Multiport Switch4/2
  Zero2/1 -> Multiport Switch2/4
  Zero7/1 -> Multiport Switch7/4
  Demux1/4 -> Multiport Switch3/3
  Demux1/5 -> Multiport Switch4/3
  Multiport Switch5/1 -> Mux/6
  Multiport Switch1/1 -> Mux/2
  Demux1/2 -> Multiport Switch1/3
  Mux/1 -> But Out/1
  Zero3/1 -> Multiport Switch3/4
  Zero1/1 -> Multiport Switch1/4
  Demux/7 -> Multiport Switch6/2
  Demux1/8 -> Multiport Switch7/3
  Multiport Switch7/1 -> Mux/8
  Demux1/6 -> Multiport Switch5/3
  Demux/3 -> Multiport Switch2/2
  Multiport Switch4/1 -> Mux/5
  Demux/1 -> Multiport Switch/2
  B1/1 -> MATLAB Function/1(A1)

== system DataPath/Subsystem1/ALU Regs/Subsystem4 ==
  Bus A1 : Inport
  A1 : Inport  Port=2
  A2 : Inport  Port=3
  Bus A2 : Inport  Port=4
  Demux : Demux  Outputs=8
  Demux1 : Demux  Outputs=8
  MATLAB Function : MATLAB Function  TreatAsAtomicUnit=on
  Multiport Switch{,1..7} (8 alike) : MultiPortSwitch  DataPortOrder=Specify indices  Inputs=2  DataPortIndices={0,1,-1}  SaturateOnIntegerOverflow=off  InputSameDT=off
  Mux : Mux  Inputs=8
  Zero{,1..7} (8 alike) : Constant  Value=0  OutDataTypeStr=Inherit: Inherit via back propagation
  But Out : Outport
  wires:
  Demux1/7 -> Multiport Switch6/3
  Multiport Switch2/1 -> Mux/3
  Demux/4 -> Multiport Switch3/2
  Bus A2/1 -> Demux1/1
  Multiport Switch6/1 -> Mux/7
  Demux1/1 -> Multiport Switch/3
  Multiport Switch3/1 -> Mux/4
  Zero/1 -> Multiport Switch/4
  MATLAB Function/1(Select) -> Multiport Switch1/1, Multiport Switch7/1, Multiport Switch6/1, Multiport Switch5/1, Multiport Switch4/1, Multiport Switch3/1, Multiport Switch2/1, Multiport Switch/1
  Demux/2 -> Multiport Switch1/2
  Demux/6 -> Multiport Switch5/2
  Demux/8 -> Multiport Switch7/2
  Multiport Switch/1 -> Mux/1
  Demux1/3 -> Multiport Switch2/3
  Zero6/1 -> Multiport Switch6/4
  Bus A1/1 -> Demux/1
  A2/1 -> MATLAB Function/2(A2)
  Zero5/1 -> Multiport Switch5/4
  Zero4/1 -> Multiport Switch4/4
  Demux/5 -> Multiport Switch4/2
  Zero2/1 -> Multiport Switch2/4
  Zero7/1 -> Multiport Switch7/4
  Demux1/4 -> Multiport Switch3/3
  Demux1/5 -> Multiport Switch4/3
  Multiport Switch5/1 -> Mux/6
  Multiport Switch1/1 -> Mux/2
  Demux1/2 -> Multiport Switch1/3
  Mux/1 -> But Out/1
  Zero3/1 -> Multiport Switch3/4
  Zero1/1 -> Multiport Switch1/4
  Demux/7 -> Multiport Switch6/2
  Demux1/8 -> Multiport Switch7/3
  Multiport Switch7/1 -> Mux/8
  Demux1/6 -> Multiport Switch5/3
  Demux/3 -> Multiport Switch2/2
  Multiport Switch4/1 -> Mux/5
  Demux/1 -> Multiport Switch/2
  A1/1 -> MATLAB Function/1(A1)

== system DataPath/Subsystem1/ALU_REG/Subsystem1 ==
  Data : Inport
  Store : Inport  Port=2
  Clock : Inport  Port=3
  Clear : Inport  Port=4
  AND : Logic  IconShape=distinctive  AllPortsSameDT=off  OutDataTypeStr=boolean
  AND1 : Logic  IconShape=distinctive  AllPortsSameDT=off  OutDataTypeStr=boolean
  D Flip-Flop : simulink_extras/Flip Flops/D Flip-Flop
  NOT : Logic  Operator=NOT  IconShape=distinctive  AllPortsSameDT=off  OutDataTypeStr=boolean
  NOT1 : Logic  Operator=NOT  IconShape=distinctive  AllPortsSameDT=off  OutDataTypeStr=boolean
  OR : Logic  Operator=OR  IconShape=distinctive  AllPortsSameDT=off  OutDataTypeStr=boolean
  Q : Outport
  !Q : Outport  Port=2
  wires:
  AND1/1 -> OR/2
  AND/1 -> OR/1
  D Flip-Flop/1 -> Q/1, AND1/2
  NOT/1 -> AND1/1
  Store/1 -> AND/2, NOT/1
  Clock/1 -> D Flip-Flop/2
  Data/1 -> AND/1
  OR/1 -> D Flip-Flop/1
  D Flip-Flop/2 -> !Q/1
  Clear/1 -> NOT1/1
  NOT1/1 -> D Flip-Flop/3

== system DataPath/Subsystem1/ALU_REG/Subsystem3 ==
  Data : Inport
  Store : Inport  Port=2
  Clock : Inport  Port=3
  Clear : Inport  Port=4
  AND : Logic  IconShape=distinctive  AllPortsSameDT=off  OutDataTypeStr=boolean
  AND1 : Logic  IconShape=distinctive  AllPortsSameDT=off  OutDataTypeStr=boolean
  D Flip-Flop : simulink_extras/Flip Flops/D Flip-Flop
  NOT : Logic  Operator=NOT  IconShape=distinctive  AllPortsSameDT=off  OutDataTypeStr=boolean
  NOT1 : Logic  Operator=NOT  IconShape=distinctive  AllPortsSameDT=off  OutDataTypeStr=boolean
  OR : Logic  Operator=OR  IconShape=distinctive  AllPortsSameDT=off  OutDataTypeStr=boolean
  Q : Outport
  !Q : Outport  Port=2
  wires:
  AND1/1 -> OR/2
  AND/1 -> OR/1
  D Flip-Flop/1 -> Q/1, AND1/2
  NOT/1 -> AND1/1
  Store/1 -> AND/2, NOT/1
  Clock/1 -> D Flip-Flop/2
  Data/1 -> AND/1
  OR/1 -> D Flip-Flop/1
  D Flip-Flop/2 -> !Q/1
  Clear/1 -> NOT1/1
  NOT1/1 -> D Flip-Flop/3

== system DataPath/Subsystem1/Add Subtract Logic/Subsystem1 ==
  AND : Inport
  OR : Inport  Port=2
  XOR : Inport  Port=3
  !A : Inport  Port=4
  "!B " : Inport  Port=5
  SR : Inport  Port=6
  SL : Inport  Port=7
  OR1 : Logic  Operator=OR  Inputs=4  IconShape=distinctive  AllPortsSameDT=off  OutDataTypeStr=boolean
  OR2 : Logic  Operator=OR  Inputs=4  IconShape=distinctive  AllPortsSameDT=off  OutDataTypeStr=boolean
  OR3 : Logic  Operator=OR  Inputs=4  IconShape=distinctive  AllPortsSameDT=off  OutDataTypeStr=boolean
  C : Outport
  B : Outport  Port=2
  "A " : Outport  Port=3
  wires:
  OR2/1 -> C/1
  OR1/1 -> B/1
  OR3/1 -> "A "/1
  OR/1 -> OR3/1
  XOR/1 -> OR3/2, OR2/3
  !A/1 -> OR3/3, OR1/3
  "!B "/1 -> OR3/4, OR1/4, OR2/4
  SR/1 -> OR2/1
  SL/1 -> OR1/1
  AND/1 -> OR1/2, OR2/2

== system DataPath/Subsystem1/Add Subtract Logic/Subsystem2 ==
  LO : Inport
  Enable : Inport  Port=2
  C : Inport  Port=3
  B : Inport  Port=4
  A : Inport  Port=5
  AND{6..17} (12 alike) : Logic  IconShape=distinctive  AllPortsSameDT=off  OutDataTypeStr=boolean
  NOT1 : Logic  Operator=NOT  IconShape=distinctive  AllPortsSameDT=off  OutDataTypeStr=boolean
  NOT2 : Logic  Operator=NOT  IconShape=distinctive  AllPortsSameDT=off  OutDataTypeStr=boolean
  NOT3 : Logic  Operator=NOT  IconShape=distinctive  AllPortsSameDT=off  OutDataTypeStr=boolean
  S-R Flip-Flop : simulink_extras/Flip Flops/S-R Flip-Flop  initial_condition=0
  S-R Flip-Flop1 : simulink_extras/Flip Flops/S-R Flip-Flop  initial_condition=0
  S-R Flip-Flop2 : simulink_extras/Flip Flops/S-R Flip-Flop  initial_condition=0
  A Stored : Outport
  B Stored : Outport  Port=2
  C Stored : Outport  Port=3
  wires:
  AND6/1 -> NOT3/1, AND14/2
  AND8/1 -> AND10/2, NOT1/1
  AND12/1 -> S-R Flip-Flop1/2
  NOT3/1 -> AND11/2
  Enable/1 -> AND8/1, AND7/1, AND6/1, AND13/1, AND12/1, AND11/1, AND10/1, AND9/1, AND14/1
  AND14/1 -> S-R Flip-Flop/1
  AND10/1 -> S-R Flip-Flop2/1
  S-R Flip-Flop1/1 -> AND16/1  "Data"
  AND7/1 -> AND9/2, NOT2/1
  AND11/1 -> S-R Flip-Flop/2
  B/1 -> AND7/2
  LO/1 -> AND17/2, AND16/2, AND15/2
  AND13/1 -> S-R Flip-Flop2/2
  AND17/1 -> C Stored/1
  A/1 -> AND6/2
  NOT2/1 -> AND12/2
  AND16/1 -> B Stored/1
  NOT1/1 -> AND13/2
  AND15/1 -> A Stored/1
  S-R Flip-Flop2/1 -> AND17/1  "Data"
  AND9/1 -> S-R Flip-Flop1/1
  S-R Flip-Flop/1 -> AND15/1  "Data"
  C/1 -> AND8/2

== system DataPath/Subsystem1/Normalize Div/Subsystem1 ==
  Data : Inport
  CLK : Inport  Port=2
  NOT9 : Logic  Operator=NOT  IconShape=distinctive  AllPortsSameDT=off  OutDataTypeStr=boolean
  Subsystem6 : Subsystem
  Subsystem7 : Subsystem
  !Q : Outport
  Q : Outport  Port=2
  wires:
  Subsystem7/1(Q) -> Subsystem6/1(Data)
  Subsystem6/1(Q) -> Q/1
  CLK/1 -> Subsystem6/2(CLK), NOT9/1
  NOT9/1 -> Subsystem7/2(CLK)
  Data/1 -> Subsystem7/1(Data)
  Subsystem6/2(!Q) -> !Q/1

== system DataPath/Subsystem1/Normalize Div/Subsystem8 ==
  Data : Inport
  CLK : Inport  Port=2
  NOT9 : Logic  Operator=NOT  IconShape=distinctive  AllPortsSameDT=off  OutDataTypeStr=boolean
  Subsystem6 : Subsystem
  Subsystem7 : Subsystem
  !Q : Outport
  Q : Outport  Port=2
  wires:
  Subsystem7/1(Q) -> Subsystem6/1(Data)
  Subsystem6/1(Q) -> Q/1
  NOT9/1 -> Subsystem7/2(CLK)
  Data/1 -> Subsystem7/1(Data)
  Subsystem6/2(!Q) -> !Q/1
  CLK/1 -> Subsystem6/2(CLK), NOT9/1

== system DataPath/Subsystem1/Stepper/Subsystem1 ==
  "Step_{n-1}" : Inport
  CLK : Inport  Port=2
  "OR_{n+1}" : Inport  Port=3
  AND1 : Logic  IconShape=distinctive  AllPortsSameDT=off  OutDataTypeStr=boolean
  DFF : Subsystem
  Delay : Delay  DelayLength=1  InputProcessing=Columns as channels (frame based)  SampleTime=1e-6
  NOT1 : Logic  Operator=NOT  IconShape=distinctive  AllPortsSameDT=off  OutDataTypeStr=boolean
  OR1 : Logic  Operator=OR  IconShape=distinctive  AllPortsSameDT=off  OutDataTypeStr=boolean
  "Step_{n}" : Outport
  "!Step_{n}" : Outport  Port=2
  "OR_{n}" : Outport  Port=3
  wires:
  NOT1/1 -> "!Step_{n}"/1, AND1/2
  CLK/1 -> DFF/2(CLK)
  AND1/1 -> DFF/1(Data)
  "OR_{n+1}"/1 -> OR1/2
  "Step_{n-1}"/1 -> AND1/1
  DFF/1(Q) -> "Step_{n}"/1, OR1/1
  OR1/1 -> Delay/1
  Delay/1 -> "OR_{n}"/1, NOT1/1

== system DataPath/Subsystem1/Stepper/Subsystem2 ==
  "Step_{n-1}" : Inport
  CLK : Inport  Port=2
  "OR_{n+1}" : Inport  Port=3
  AND1 : Logic  IconShape=distinctive  AllPortsSameDT=off  OutDataTypeStr=boolean
  DFF : Subsystem
  Delay : Delay  DelayLength=1  InputProcessing=Columns as channels (frame based)  SampleTime=1e-6
  Delay One Step : Delay  DelayLength=1
  Delay One Step1 : Delay  DelayLength=1
  NOT1 : Logic  Operator=NOT  IconShape=distinctive  AllPortsSameDT=off  OutDataTypeStr=boolean
  OR1 : Logic  Operator=OR  IconShape=distinctive  AllPortsSameDT=off  OutDataTypeStr=boolean
  "Step_{n}" : Outport
  "!Step_{n}" : Outport  Port=2
  "OR_{n}" : Outport  Port=3
  wires:
  Delay One Step1/1 -> "!Step_{n}"/1, AND1/2
  CLK/1 -> DFF/2(CLK)
  AND1/1 -> DFF/1(Data)
  "OR_{n+1}"/1 -> OR1/2
  "Step_{n-1}"/1 -> AND1/1
  DFF/1(Q) -> "Step_{n}"/1, OR1/1
  OR1/1 -> Delay/1
  Delay/1 -> Delay One Step/1, NOT1/1
  Delay One Step/1 -> "OR_{n}"/1
  NOT1/1 -> Delay One Step1/1

== system DataPath/Subsystem1/Stepper/Subsystem3 ==
  "Step_{n-1}" : Inport
  CLK : Inport  Port=2
  "OR_{n+1}" : Inport  Port=3
  AND1 : Logic  IconShape=distinctive  AllPortsSameDT=off  OutDataTypeStr=boolean
  DFF : Subsystem
  Delay : Delay  DelayLength=1  InputProcessing=Columns as channels (frame based)  SampleTime=1e-6
  NOT1 : Logic  Operator=NOT  IconShape=distinctive  AllPortsSameDT=off  OutDataTypeStr=boolean
  OR1 : Logic  Operator=OR  IconShape=distinctive  AllPortsSameDT=off  OutDataTypeStr=boolean
  "Step_{n}" : Outport
  "!Step_{n}" : Outport  Port=2
  "OR_{n}" : Outport  Port=3
  wires:
  NOT1/1 -> "!Step_{n}"/1, AND1/2
  CLK/1 -> DFF/2(CLK)
  AND1/1 -> DFF/1(Data)
  "OR_{n+1}"/1 -> OR1/2
  "Step_{n-1}"/1 -> AND1/1
  DFF/1(Q) -> "Step_{n}"/1, OR1/1
  OR1/1 -> Delay/1
  Delay/1 -> "OR_{n}"/1, NOT1/1

== system DataPath/Subsystem1/Stepper/Subsystem4 ==
  "Step_{n-1}" : Inport
  CLK : Inport  Port=2
  "OR_{n+1}" : Inport  Port=3
  AND1 : Logic  IconShape=distinctive  AllPortsSameDT=off  OutDataTypeStr=boolean
  DFF : Subsystem
  Delay : Delay  DelayLength=1  InputProcessing=Columns as channels (frame based)  SampleTime=1e-6
  NOT1 : Logic  Operator=NOT  IconShape=distinctive  AllPortsSameDT=off  OutDataTypeStr=boolean
  OR1 : Logic  Operator=OR  IconShape=distinctive  AllPortsSameDT=off  OutDataTypeStr=boolean
  "Step_{n}" : Outport
  "!Step_{n}" : Outport  Port=2
  "OR_{n}" : Outport  Port=3
  wires:
  NOT1/1 -> "!Step_{n}"/1, AND1/2
  CLK/1 -> DFF/2(CLK)
  AND1/1 -> DFF/1(Data)
  "OR_{n+1}"/1 -> OR1/2
  "Step_{n-1}"/1 -> AND1/1
  DFF/1(Q) -> "Step_{n}"/1, OR1/1
  OR1/1 -> Delay/1
  Delay/1 -> "OR_{n}"/1, NOT1/1

== system DataPath/Subsystem1/Subsystem1/Subsystem ==
  Out A1-LO : Inport
  Out A1-Mult : Inport  Port=2
  Out A1-CD : Inport  Port=3
  Out A1-ND : Inport  Port=4
  Out A1-SDR : Inport  Port=5
  OR : Logic  Operator=OR  Inputs=5  IconShape=distinctive  AllPortsSameDT=off  OutDataTypeStr=boolean
  Out A1 : Outport
  wires:
  Out A1-LO/1 -> OR/5
  Out A1-Mult/1 -> OR/1
  OR/1 -> Out A1/1  "Out A1"
  Out A1-CD/1 -> OR/2
  Out A1-ND/1 -> OR/3
  Out A1-SDR/1 -> OR/4

== system DataPath/Subsystem1/Subsystem1/Subsystem10 ==
  LSB-Mult : Inport
  LSB-CD : Inport  Port=2
  OR2 : Logic  Operator=OR  IconShape=distinctive  AllPortsSameDT=off  OutDataTypeStr=boolean
  LSB : Outport
  wires:
  LSB-CD/1 -> OR2/1
  LSB-Mult/1 -> OR2/2
  OR2/1 -> LSB/1  "LSB"

== system DataPath/Subsystem1/Subsystem1/Subsystem11 ==
  NegA-ND : Inport
  NegA-SDR : Inport  Port=2
  OR1 : Logic  Operator=OR  IconShape=distinctive  AllPortsSameDT=off  OutDataTypeStr=boolean
  NegA : Outport
  wires:
  NegA-ND/1 -> OR1/1
  NegA-SDR/1 -> OR1/2
  OR1/1 -> NegA/1  "Bus Switch"

== system DataPath/Subsystem1/Subsystem1/Subsystem13 ==
  Store B2-Mult : Inport
  Store B2-CD : Inport  Port=2
  Store B2-SDR : Inport  Port=3
  CLR : Inport  Port=4
  OR2 : Logic  Operator=OR  Inputs=4  IconShape=distinctive  AllPortsSameDT=off  OutDataTypeStr=boolean
  Store B2 : Outport
  wires:
  Store B2-CD/1 -> OR2/2
  OR2/1 -> Store B2/1  "Store B2"
  Store B2-SDR/1 -> OR2/3
  Store B2-Mult/1 -> OR2/1
  CLR/1 -> OR2/4

== system DataPath/Subsystem1/Subsystem1/Subsystem14 ==
  Store B1-ICS : Inport
  Store B1-Mult : Inport  Port=2
  Store B1-ND : Inport  Port=3
  In4 : Inport  Port=4
  OR1 : Logic  Operator=OR  Inputs=4  IconShape=distinctive  AllPortsSameDT=off  OutDataTypeStr=boolean
  Store B1 : Outport
  wires:
  Store B1-ND/1 -> OR1/2
  Store B1-ICS/1 -> OR1/1
  OR1/1 -> Store B1/1  "Store B1"
  Store B1-Mult/1 -> OR1/3
  In4/1 -> OR1/4

== system DataPath/Subsystem1/Subsystem1/Subsystem2 ==
  Out B2-Mult : Inport
  Out B2-CD : Inport  Port=2
  Out B2-SDR : Inport  Port=3
  OR2 : Logic  Operator=OR  Inputs=3  IconShape=distinctive  AllPortsSameDT=off  OutDataTypeStr=boolean
  Out B2 : Outport
  wires:
  Out B2-Mult/1 -> OR2/1
  Out B2-CD/1 -> OR2/2
  Out B2-SDR/1 -> OR2/3
  OR2/1 -> Out B2/1  "Out B2"

== system DataPath/Subsystem1/Subsystem1/Subsystem3 ==
  Out ALU-LO : Inport
  Out ALU-Mult : Inport  Port=2
  Out ALU-ND : Inport  Port=3
  Out ALU-CD : Inport  Port=4
  Out ALU-SDR : Inport  Port=5
  OR3 : Logic  Operator=OR  Inputs=5  IconShape=distinctive  AllPortsSameDT=off  OutDataTypeStr=boolean
  Out ALU : Outport
  wires:
  Out ALU-SDR/1 -> OR3/4
  Out ALU-Mult/1 -> OR3/1
  OR3/1 -> Out ALU/1  "Out A1"
  Out ALU-LO/1 -> OR3/5
  Out ALU-ND/1 -> OR3/3
  Out ALU-CD/1 -> OR3/2

== system DataPath/Subsystem1/Subsystem1/Subsystem5 ==
  Out B1-LO : Inport
  Out B1-mult : Inport  Port=2
  Out B1-CD : Inport  Port=3
  Out B1-ND : Inport  Port=4
  OR1 : Logic  Operator=OR  Inputs=4  IconShape=distinctive  AllPortsSameDT=off  OutDataTypeStr=boolean
  Out B1 : Outport
  wires:
  Out B1-CD/1 -> OR1/2
  Out B1-mult/1 -> OR1/1
  Out B1-LO/1 -> OR1/4
  OR1/1 -> Out B1/1  "Out B1"
  Out B1-ND/1 -> OR1/3
